simulink model "Target_Control_System"  (R2021b)
settings: Solver=FixedStepDiscrete  StartTime=0.0  StopTime=5  RelTol=1e-3
PreLoadFcn:
  | RTWConfigurationCB('preloadfcn', bdroot);
PostLoadFcn:
  | load('configuration/data_struct.mat');
  | load('configuration/fluxMaps_propMotor.mat');
  | load('configuration/parameterInit_PROP.mat');
  | load('configuration/parameterInit_PUMP.mat');
  | load('configuration/parameterInit_PITCH.mat');
  | load('configuration/parameterInit_TILT.mat');
  | %load('configuration/base_workspace_signal_definition.mat');
  | %load('resolvedatastores_to_baseworkspace_for_faster_simulation.mat');
model workspace (MAT data in the model file):
  SIMULATION_OPTIONS : Simulink.Parameter (value not decoded)
  TARGET_CODE_GEN : Simulink.Parameter (value not decoded)
  TCS_SAMPLE_FREQ_HZ : Simulink.Parameter (value not decoded)
symbols that are objects in the model workspace (value not decoded): TARGET_CODE_GEN, TCS_SAMPLE_FREQ_HZ
undefined symbols (not defined in the file): A_DQ_REF_LPF_INIT__PITCH, A_DQ_REF_LPF_INIT__PROP, A_DQ_REF_LPF_INIT__PUMP, A_DQ_REF_LPF_INIT__TILT, A_OBSERVER_CONFIDENCE_INIT__PITCH, A_OBSERVER_CONFIDENCE_INIT__PROP, A_OBSERVER_CONFIDENCE_INIT__PUMP, A_OBSERVER_CONFIDENCE_INIT__TILT, ACTUATOR_MAX_ANGLE_TRIP__PITCH, ACTUATOR_MIN_ANGLE_TRIP__PITCH, ACTUATOR_POS_SENSOR_INV_DIRECTION__PITCH, ACTUATOR_POS_SENSOR_INV_DIRECTION__TILT, ACTUATOR_POS_SENSOR_OFFSET__PITCH, ACTUATOR_POS_SENSOR_OFFSET__TILT, ADC_scaler1_baseaddr_TILT, ADC_SCALER_FLOAT_TO_FIXPOINT_EXPANSION, ANGLE_ELEC_FROM_SENSOR_OFFSET_INIT__PITCH, ANGLE_ELEC_FROM_SENSOR_OFFSET_INIT__PROP, ANGLE_ELEC_FROM_SENSOR_OFFSET_INIT__PUMP, ANGLE_ELEC_FROM_SENSOR_OFFSET_INIT__TILT, AUTO_CLEAR_FAULTS_ENABLED__PITCH, AUTO_CLEAR_FAULTS_ENABLED__PROP, AUTO_CLEAR_FAULTS_ENABLED__PUMP, AUTO_CLEAR_FAULTS_ENABLED__TILT, AUTO_CLEAR_FAULTS_WAIT_TICKS__PITCH, AUTO_CLEAR_FAULTS_WAIT_TICKS__PROP, AUTO_CLEAR_FAULTS_WAIT_TICKS__PUMP, AUTO_CLEAR_FAULTS_WAIT_TICKS__TILT, AUTO_I_ZERO_IDLE_TICKS__PITCH, AUTO_I_ZERO_IDLE_TICKS__PROP, AUTO_I_ZERO_IDLE_TICKS__PUMP, AUTO_I_ZERO_IDLE_TICKS__TILT, AUTO_I_ZERO_OFFSET_IDC_THRESHOLD__PITCH, AUTO_I_ZERO_OFFSET_IDC_THRESHOLD__PROP, AUTO_I_ZERO_OFFSET_IDC_THRESHOLD__PUMP, AUTO_I_ZERO_OFFSET_IDC_THRESHOLD__TILT, AUTO_I_ZERO_OFFSET_IPH_THRESHOLD__PITCH, AUTO_I_ZERO_OFFSET_IPH_THRESHOLD__PROP, AUTO_I_ZERO_OFFSET_IPH_THRESHOLD__PUMP, AUTO_I_ZERO_OFFSET_IPH_THRESHOLD__TILT, AUTO_SENSORLESS_SWITCHOVER_DISABLE_OMEGA, AUTO_SENSORLESS_SWITCHOVER_ENABLE_OMEGA, AUTO_SENSORLESS_SWITCHOVER_MIN_CONFIDENCE, AUXILIARY_PROTECTION_UNIT_BASEADDR__TILT, blanking_max_error_omega_INIT_PITCH, blanking_max_error_omega_INIT_TILT, blanking_max_error_position_INIT_PITCH, blanking_max_error_position_INIT_TILT, BRUTE_START_I_Q_REF_RAMP_SPEED__PITCH, BRUTE_START_I_Q_REF_RAMP_SPEED__PROP, BRUTE_START_I_Q_REF_RAMP_SPEED__PUMP, BRUTE_START_I_Q_REF_RAMP_SPEED__TILT, CONTROL_LOOP_DT_INIT__PITCH, CONTROL_LOOP_DT_INIT__PROP, CONTROL_LOOP_DT_INIT__PUMP, CONTROL_LOOP_DT_INIT__TILT, CORRECTION_FILTER_SCALE__PITCH, CORRECTION_FILTER_SCALE__PROP, CORRECTION_FILTER_SCALE__PUMP, CORRECTION_FILTER_SCALE__TILT ... (+458)
libraries: simulink x178, Reusables_Lib x24
(part 24 of 47)

== system Target_Control_System/Target_Control_System/Simulation Controls/Simulation Data Store Initialization/setupIirFilters(&oTilt)/computeCoefficientsButter()1 ==
  fCutoffFrequencyHz : Inport  OutDataTypeStr=single
  dSampleFrequencyHz : Inport  Port=2  OutDataTypeStr=single
  Add : Sum  Inputs=+++  OutDataTypeStr=double
  Add1 : Sum  Inputs=-+
  Add2 : Sum  Inputs=+-+  OutDataTypeStr=double
  Constant : Constant  Value=0.0008  OutDataTypeStr=single  SampleTime=-1
  Constant1 : Constant  Value=0.45  OutDataTypeStr=single  SampleTime=-1
  Constant{5,7,9..10} (4 alike) : Constant  SampleTime=-1
  Constant2 : Constant  Value=pi  OutDataTypeStr=double  SampleTime=-1
  Constant3 : Constant  OutDataTypeStr=double  SampleTime=-1
  Constant4 : Constant  Value=sqrt(2)  OutDataTypeStr=double  SampleTime=-1
  Constant6 : Constant  OutDataTypeStr=double  SampleTime=-1
  Constant8 : Constant  Value=2  SampleTime=-1
  Data Type Conversion : DataTypeConversion  OutDataTypeStr=double
  Divide : Product  Inputs=**  OutDataTypeStr=single
  Divide1 : Product  Inputs=**  OutDataTypeStr=single
  Divide{3,5..6,8,10..11} (6 alike) : Product  Inputs=**  OutDataTypeStr=double
  Divide2 : Product  Inputs=*/  OutDataTypeStr=double
  Divide4 : Product  Inputs=*/  OutDataTypeStr=double
  Divide7 : Product  Inputs=*/  OutDataTypeStr=double
  Divide9 : Product  Inputs=***  OutDataTypeStr=double
  Gain : Gain  Gain=2  OutDataTypeStr=double
  Gain1 : Gain  Gain=-1  OutDataTypeStr=double
  Gain2 : Gain  Gain=-1  OutDataTypeStr=double
  Gain3 : Gain  Gain=-1  OutDataTypeStr=double
  Mux : Mux  Inputs=6
  Saturation Dynamic : simulink/Discontinuities/Saturation Dynamic  OutMin=[]  OutMax=[]  OutDataTypeStr=Inherit: Same as second input  OutDataType=fixdt(1, 16)  OutScaling=2^-10  DoSatur=off
  Tan : Trigonometry  Operator=tan
  dpOutArray : Outport
  fCutoffFrequencyHz_out : Outport  Port=2
  wires:
  Saturation Dynamic/1 -> Data Type Conversion/1, fCutoffFrequencyHz_out/1  "fCutoffFrequencyHz"
  Data Type Conversion/1 -> Divide2/1
  Constant10/1 -> Mux/4
  [dA2] -> Gain3/1
  Gain3/1 -> Mux/6
  [dA1] -> Gain2/1
  Gain2/1 -> Mux/5
  [dB2] -> Mux/3
  [dB1] -> Mux/2
  [dB0] -> Mux/1
  Divide11/1 -> [dA2]
  Gain1/1 -> Divide11/2
  Add2/1 -> Gain1/1
  Constant9/1 -> Add2/3
  Divide10/1 -> Add2/2
  [kdQ] -> Divide10/2
  Constant7/1 -> Add1/1
  Divide8/1 -> Add1/2, Add2/1
  Divide9/1 -> [dA1]
  Constant8/1 -> Divide9/3
  Add1/1 -> Divide9/2
  [kdIta] -> Divide8/1, Divide8/2, Divide10/1
  Gain/1 -> [dB1]
  Divide7/1 -> [dB0], Gain/1, [dB2], Divide9/1, Divide11/1
  Add/1 -> Divide7/2
  Constant6/1 -> Divide7/1
  Constant5/1 -> Add/3
  Divide5/1 -> Add/2
  Divide6/1 -> Add/1
  [kdQ] -> Divide5/2
  [kdIta] -> Divide5/1, Divide6/1, Divide6/2
  Mux/1 -> dpOutArray/1
  Constant4/1 -> [kdQ]
  Divide4/1 -> [kdIta]
  Constant3/1 -> Divide4/1
  Tan/1 -> Divide4/2
  Divide3/1 -> Tan/1
  Constant2/1 -> Divide3/2
  Divide2/1 -> Divide3/1  "dFf"
  Constant/1 -> Divide/2
  fCutoffFrequencyHz/1 -> Saturation Dynamic/2  "fCutoffFrequencyHz"
  Divide1/1 -> Saturation Dynamic/1
  dSampleFrequencyHz/1 -> Divide1/2, Divide2/2, Divide/1
  Constant1/1 -> Divide1/1
  Divide/1 -> Saturation Dynamic/3

== system Target_Control_System/Target_Control_System/Simulation Controls/Simulation Data Store Initialization/setupIirFilters(&oTilt)/computeCoefficientsButter()2 ==
  fCutoffFrequencyHz : Inport  OutDataTypeStr=single
  dSampleFrequencyHz : Inport  Port=2  OutDataTypeStr=single
  Add : Sum  Inputs=+++  OutDataTypeStr=double
  Add1 : Sum  Inputs=-+
  Add2 : Sum  Inputs=+-+  OutDataTypeStr=double
  Constant : Constant  Value=0.0008  OutDataTypeStr=single  SampleTime=-1
  Constant1 : Constant  Value=0.45  OutDataTypeStr=single  SampleTime=-1
  Constant{5,7,9..10} (4 alike) : Constant  SampleTime=-1
  Constant2 : Constant  Value=pi  OutDataTypeStr=double  SampleTime=-1
  Constant3 : Constant  OutDataTypeStr=double  SampleTime=-1
  Constant4 : Constant  Value=sqrt(2)  OutDataTypeStr=double  SampleTime=-1
  Constant6 : Constant  OutDataTypeStr=double  SampleTime=-1
  Constant8 : Constant  Value=2  SampleTime=-1
  Data Type Conversion : DataTypeConversion  OutDataTypeStr=double
  Divide : Product  Inputs=**  OutDataTypeStr=single
  Divide1 : Product  Inputs=**  OutDataTypeStr=single
  Divide{3,5..6,8,10..11} (6 alike) : Product  Inputs=**  OutDataTypeStr=double
  Divide2 : Product  Inputs=*/  OutDataTypeStr=double
  Divide4 : Product  Inputs=*/  OutDataTypeStr=double
  Divide7 : Product  Inputs=*/  OutDataTypeStr=double
  Divide9 : Product  Inputs=***  OutDataTypeStr=double
  Gain : Gain  Gain=2  OutDataTypeStr=double
  Gain1 : Gain  Gain=-1  OutDataTypeStr=double
  Gain2 : Gain  Gain=-1  OutDataTypeStr=double
  Gain3 : Gain  Gain=-1  OutDataTypeStr=double
  Mux : Mux  Inputs=6
  Saturation Dynamic : simulink/Discontinuities/Saturation Dynamic  OutMin=[]  OutMax=[]  OutDataTypeStr=Inherit: Same as second input  OutDataType=fixdt(1, 16)  OutScaling=2^-10  DoSatur=off
  Tan : Trigonometry  Operator=tan
  dpOutArray : Outport
  fCutoffFrequencyHz_out : Outport  Port=2
  wires:
  Saturation Dynamic/1 -> Data Type Conversion/1, fCutoffFrequencyHz_out/1  "fCutoffFrequencyHz"
  Data Type Conversion/1 -> Divide2/1
  Constant10/1 -> Mux/4
  [dA2] -> Gain3/1
  Gain3/1 -> Mux/6
  [dA1] -> Gain2/1
  Gain2/1 -> Mux/5
  [dB2] -> Mux/3
  [dB1] -> Mux/2
  [dB0] -> Mux/1
  Divide11/1 -> [dA2]
  Gain1/1 -> Divide11/2
  Add2/1 -> Gain1/1
  Constant9/1 -> Add2/3
  Divide10/1 -> Add2/2
  [kdQ] -> Divide10/2
  Constant7/1 -> Add1/1
  Divide8/1 -> Add1/2, Add2/1
  Divide9/1 -> [dA1]
  Constant8/1 -> Divide9/3
  Add1/1 -> Divide9/2
  [kdIta] -> Divide8/1, Divide8/2, Divide10/1
  Gain/1 -> [dB1]
  Divide7/1 -> [dB0], Gain/1, [dB2], Divide9/1, Divide11/1
  Add/1 -> Divide7/2
  Constant6/1 -> Divide7/1
  Constant5/1 -> Add/3
  Divide5/1 -> Add/2
  Divide6/1 -> Add/1
  [kdQ] -> Divide5/2
  [kdIta] -> Divide5/1, Divide6/1, Divide6/2
  Mux/1 -> dpOutArray/1
  Constant4/1 -> [kdQ]
  Divide4/1 -> [kdIta]
  Constant3/1 -> Divide4/1
  Tan/1 -> Divide4/2
  Divide3/1 -> Tan/1
  Constant2/1 -> Divide3/2
  Divide2/1 -> Divide3/1  "dFf"
  Constant/1 -> Divide/2
  fCutoffFrequencyHz/1 -> Saturation Dynamic/2  "fCutoffFrequencyHz"
  Divide1/1 -> Saturation Dynamic/1
  dSampleFrequencyHz/1 -> Divide1/2, Divide2/2, Divide/1
  Constant1/1 -> Divide1/1
  Divide/1 -> Saturation Dynamic/3

== system Target_Control_System/Target_Control_System/Simulation Controls/Simulation Data Store Initialization/setupIirFilters(&oTilt)/softwareIirFilterInitialize() ==
  fFreq3db : Inport
  fFreqSample : Inport  Port=2
  Constant : Constant  OutDataTypeStr=single  SampleTime=-1
  Constant1 : Constant  Value=0  OutDataTypeStr=single  SampleTime=-1
  Data Store Write : DataStoreWrite  DataStoreName=oTilt  DataStoreElements=oTilt.oMot_.oState_.oMotorAccelerationFilterStage2_.afConstantsA_.h0  IndexOptions=Index vector (dialog)  Indices=1  OutputSizes=1
  Data Store Write1 : DataStoreWrite  DataStoreName=oTilt  DataStoreElements=oTilt.oMot_.oState_.oMotorAccelerationFilterStage2_.afConstantsA_.h1  IndexOptions=Index vector (dialog)  Indices=1  OutputSizes=1
  Data Store Write10 : DataStoreWrite  DataStoreName=oTilt  DataStoreElements=oTilt.oMot_.oState_.oMotorAccelerationFilterStage2_.fFilterOutput_  IndexOptions=Index vector (dialog)  Indices=1  OutputSizes=1
  Data Store Write2 : DataStoreWrite  DataStoreName=oTilt  DataStoreElements=oTilt.oMot_.oState_.oMotorAccelerationFilterStage2_.afConstantsA_.h2  IndexOptions=Index vector (dialog)  Indices=1  OutputSizes=1
  Data Store Write3 : DataStoreWrite  DataStoreName=oTilt  DataStoreElements=oTilt.oMot_.oState_.oMotorAccelerationFilterStage2_.afConstantsB_.h2  IndexOptions=Index vector (dialog)  Indices=1  OutputSizes=1
  Data Store Write4 : DataStoreWrite  DataStoreName=oTilt  DataStoreElements=oTilt.oMot_.oState_.oMotorAccelerationFilterStage2_.afConstantsB_.h1  IndexOptions=Index vector (dialog)  Indices=1  OutputSizes=1
  Data Store Write5 : DataStoreWrite  DataStoreName=oTilt  DataStoreElements=oTilt.oMot_.oState_.oMotorAccelerationFilterStage2_.afConstantsB_.h0  IndexOptions=Index vector (dialog)  Indices=1  OutputSizes=1
  Data Store Write6 : DataStoreWrite  DataStoreName=oTilt  DataStoreElements=oTilt.oMot_.oState_.oMotorAccelerationFilterStage2_.afPreviousInputs_.h0  IndexOptions=Index vector (dialog)  Indices=1  OutputSizes=1
  Data Store Write7 : DataStoreWrite  DataStoreName=oTilt  DataStoreElements=oTilt.oMot_.oState_.oMotorAccelerationFilterStage2_.afPreviousInputs_.h1  IndexOptions=Index vector (dialog)  Indices=1  OutputSizes=1
  Data Store Write8 : DataStoreWrite  DataStoreName=oTilt  DataStoreElements=oTilt.oMot_.oState_.oMotorAccelerationFilterStage2_.afPreviousOutputs_.h0  IndexOptions=Index vector (dialog)  Indices=1  OutputSizes=1
  Data Store Write9 : DataStoreWrite  DataStoreName=oTilt  DataStoreElements=oTilt.oMot_.oState_.oMotorAccelerationFilterStage2_.afPreviousOutputs_.h1  IndexOptions=Index vector (dialog)  Indices=1  OutputSizes=1
  Data Type Conversion{1..5} (5 alike) : DataTypeConversion  OutDataTypeStr=single
  Demux : Demux  Outputs=6
  Divide : Product  Inputs=*/  OutDataTypeStr=single
  computeCoefficientsButter() : Subsystem
  fActualFrequencyHz : Outport
  wires:
  Data Type Conversion5/1 -> Data Store Write2/1
  Data Type Conversion4/1 -> Data Store Write1/1
  Data Type Conversion3/1 -> Data Store Write3/1
  Data Type Conversion1/1 -> Data Store Write4/1
  Data Type Conversion2/1 -> Data Store Write5/1
  fFreqSample/1 -> computeCoefficientsButter()/2(dSampleFrequencyHz)
  Constant1/1 -> Data Store Write6/1, Data Store Write7/1, Data Store Write9/1, Data Store Write10/1, Data Store Write8/1
  Demux/1 -> Data Type Conversion2/1
  Demux/2 -> Data Type Conversion1/1
  Constant/1 -> Divide/1
  Divide/1 -> Data Store Write/1
  Demux/4 -> Divide/2
  Demux/3 -> Data Type Conversion3/1
  Demux/5 -> Data Type Conversion4/1
  Demux/6 -> Data Type Conversion5/1
  computeCoefficientsButter()/1(dpOutArray) -> Demux/1
  fFreq3db/1 -> computeCoefficientsButter()/1(fCutoffFrequencyHz)
  computeCoefficientsButter()/2(fFreq3db) -> fActualFrequencyHz/1

== system Target_Control_System/Target_Control_System/Simulation Controls/Simulation Data Store Initialization/setupIirFilters()/computeCoefficientsButter() ==
  fCutoffFrequencyHz : Inport  OutDataTypeStr=single
  dSampleFrequencyHz : Inport  Port=2  OutDataTypeStr=single
  Add : Sum  Inputs=+++  OutDataTypeStr=double
  Add1 : Sum  Inputs=-+
  Add2 : Sum  Inputs=+-+  OutDataTypeStr=double
  Constant : Constant  Value=0.0008  OutDataTypeStr=single  SampleTime=-1
  Constant1 : Constant  Value=0.45  OutDataTypeStr=single  SampleTime=-1
  Constant{5,7,9..10} (4 alike) : Constant  SampleTime=-1
  Constant2 : Constant  Value=pi  OutDataTypeStr=double  SampleTime=-1
  Constant3 : Constant  OutDataTypeStr=double  SampleTime=-1
  Constant4 : Constant  Value=sqrt(2)  OutDataTypeStr=double  SampleTime=-1
  Constant6 : Constant  OutDataTypeStr=double  SampleTime=-1
  Constant8 : Constant  Value=2  SampleTime=-1
  Data Type Conversion : DataTypeConversion  OutDataTypeStr=double
  Divide : Product  Inputs=**  OutDataTypeStr=single
  Divide1 : Product  Inputs=**  OutDataTypeStr=single
  Divide{3,5..6,8,10..11} (6 alike) : Product  Inputs=**  OutDataTypeStr=double
  Divide2 : Product  Inputs=*/  OutDataTypeStr=double
  Divide4 : Product  Inputs=*/  OutDataTypeStr=double
  Divide7 : Product  Inputs=*/  OutDataTypeStr=double
  Divide9 : Product  Inputs=***  OutDataTypeStr=double
  Gain : Gain  Gain=2  OutDataTypeStr=double
  Gain1 : Gain  Gain=-1  OutDataTypeStr=double
  Gain2 : Gain  Gain=-1  OutDataTypeStr=double
  Gain3 : Gain  Gain=-1  OutDataTypeStr=double
  Mux : Mux  Inputs=6
  Saturation Dynamic : simulink/Discontinuities/Saturation Dynamic  OutMin=[]  OutMax=[]  OutDataTypeStr=Inherit: Same as second input  OutDataType=fixdt(1, 16)  OutScaling=2^-10  DoSatur=off
  Tan : Trigonometry  Operator=tan
  dpOutArray : Outport
  fCutoffFrequencyHz_out : Outport  Port=2
  wires:
  Saturation Dynamic/1 -> Data Type Conversion/1, fCutoffFrequencyHz_out/1  "fCutoffFrequencyHz"
  Data Type Conversion/1 -> Divide2/1
  Constant10/1 -> Mux/4
  [dA2] -> Gain3/1
  Gain3/1 -> Mux/6
  [dA1] -> Gain2/1
  Gain2/1 -> Mux/5
  [dB2] -> Mux/3
  [dB1] -> Mux/2
  [dB0] -> Mux/1
  Divide11/1 -> [dA2]
  Gain1/1 -> Divide11/2
  Add2/1 -> Gain1/1
  Constant9/1 -> Add2/3
  Divide10/1 -> Add2/2
  [kdQ] -> Divide10/2
  Constant7/1 -> Add1/1
  Divide8/1 -> Add1/2, Add2/1
  Divide9/1 -> [dA1]
  Constant8/1 -> Divide9/3
  Add1/1 -> Divide9/2
  [kdIta] -> Divide8/1, Divide8/2, Divide10/1
  Gain/1 -> [dB1]
  Divide7/1 -> [dB0], Gain/1, [dB2], Divide9/1, Divide11/1
  Add/1 -> Divide7/2
  Constant6/1 -> Divide7/1
  Constant5/1 -> Add/3
  Divide5/1 -> Add/2
  Divide6/1 -> Add/1
  [kdQ] -> Divide5/2
  [kdIta] -> Divide5/1, Divide6/1, Divide6/2
  Mux/1 -> dpOutArray/1
  Constant4/1 -> [kdQ]
  Divide4/1 -> [kdIta]
  Constant3/1 -> Divide4/1
  Tan/1 -> Divide4/2
  Divide3/1 -> Tan/1
  Constant2/1 -> Divide3/2
  Divide2/1 -> Divide3/1  "dFf"
  Constant/1 -> Divide/2
  fCutoffFrequencyHz/1 -> Saturation Dynamic/2  "fCutoffFrequencyHz"
  Divide1/1 -> Saturation Dynamic/1
  dSampleFrequencyHz/1 -> Divide1/2, Divide2/2, Divide/1
  Constant1/1 -> Divide1/1
  Divide/1 -> Saturation Dynamic/3

== system Target_Control_System/Target_Control_System/Simulation Controls/Simulation Data Store Initialization/setupIirFilters()/computeCoefficientsButter()1 ==
  fCutoffFrequencyHz : Inport  OutDataTypeStr=single
  dSampleFrequencyHz : Inport  Port=2  OutDataTypeStr=single
  Add : Sum  Inputs=+++  OutDataTypeStr=double
  Add1 : Sum  Inputs=-+
  Add2 : Sum  Inputs=+-+  OutDataTypeStr=double
  Constant : Constant  Value=0.0008  OutDataTypeStr=single  SampleTime=-1
  Constant1 : Constant  Value=0.45  OutDataTypeStr=single  SampleTime=-1
  Constant{5,7,9..10} (4 alike) : Constant  SampleTime=-1
  Constant2 : Constant  Value=pi  OutDataTypeStr=double  SampleTime=-1
  Constant3 : Constant  OutDataTypeStr=double  SampleTime=-1
  Constant4 : Constant  Value=sqrt(2)  OutDataTypeStr=double  SampleTime=-1
  Constant6 : Constant  OutDataTypeStr=double  SampleTime=-1
  Constant8 : Constant  Value=2  SampleTime=-1
  Data Type Conversion : DataTypeConversion  OutDataTypeStr=double
  Divide : Product  Inputs=**  OutDataTypeStr=single
  Divide1 : Product  Inputs=**  OutDataTypeStr=single
  Divide{3,5..6,8,10..11} (6 alike) : Product  Inputs=**  OutDataTypeStr=double
  Divide2 : Product  Inputs=*/  OutDataTypeStr=double
  Divide4 : Product  Inputs=*/  OutDataTypeStr=double
  Divide7 : Product  Inputs=*/  OutDataTypeStr=double
  Divide9 : Product  Inputs=***  OutDataTypeStr=double
  Gain : Gain  Gain=2  OutDataTypeStr=double
  Gain1 : Gain  Gain=-1  OutDataTypeStr=double
  Gain2 : Gain  Gain=-1  OutDataTypeStr=double
  Gain3 : Gain  Gain=-1  OutDataTypeStr=double
  Mux : Mux  Inputs=6
  Saturation Dynamic : simulink/Discontinuities/Saturation Dynamic  OutMin=[]  OutMax=[]  OutDataTypeStr=Inherit: Same as second input  OutDataType=fixdt(1, 16)  OutScaling=2^-10  DoSatur=off
  Tan : Trigonometry  Operator=tan
  dpOutArray : Outport
  fCutoffFrequencyHz_out : Outport  Port=2
  wires:
  Saturation Dynamic/1 -> Data Type Conversion/1, fCutoffFrequencyHz_out/1  "fCutoffFrequencyHz"
  Data Type Conversion/1 -> Divide2/1
  Constant10/1 -> Mux/4
  [dA2] -> Gain3/1
  Gain3/1 -> Mux/6
  [dA1] -> Gain2/1
  Gain2/1 -> Mux/5
  [dB2] -> Mux/3
  [dB1] -> Mux/2
  [dB0] -> Mux/1
  Divide11/1 -> [dA2]
  Gain1/1 -> Divide11/2
  Add2/1 -> Gain1/1
  Constant9/1 -> Add2/3
  Divide10/1 -> Add2/2
  [kdQ] -> Divide10/2
  Constant7/1 -> Add1/1
  Divide8/1 -> Add1/2, Add2/1
  Divide9/1 -> [dA1]
  Constant8/1 -> Divide9/3
  Add1/1 -> Divide9/2
  [kdIta] -> Divide8/1, Divide8/2, Divide10/1
  Gain/1 -> [dB1]
  Divide7/1 -> [dB0], Gain/1, [dB2], Divide9/1, Divide11/1
  Add/1 -> Divide7/2
  Constant6/1 -> Divide7/1
  Constant5/1 -> Add/3
  Divide5/1 -> Add/2
  Divide6/1 -> Add/1
  [kdQ] -> Divide5/2
  [kdIta] -> Divide5/1, Divide6/1, Divide6/2
  Mux/1 -> dpOutArray/1
  Constant4/1 -> [kdQ]
  Divide4/1 -> [kdIta]
  Constant3/1 -> Divide4/1
  Tan/1 -> Divide4/2
  Divide3/1 -> Tan/1
  Constant2/1 -> Divide3/2
  Divide2/1 -> Divide3/1  "dFf"
  Constant/1 -> Divide/2
  fCutoffFrequencyHz/1 -> Saturation Dynamic/2  "fCutoffFrequencyHz"
  Divide1/1 -> Saturation Dynamic/1
  dSampleFrequencyHz/1 -> Divide1/2, Divide2/2, Divide/1
  Constant1/1 -> Divide1/1
  Divide/1 -> Saturation Dynamic/3

== system Target_Control_System/Target_Control_System/Simulation Controls/Simulation Data Store Initialization/setupIirFilters()/computeCoefficientsButter()2 ==
  fCutoffFrequencyHz : Inport  OutDataTypeStr=single
  dSampleFrequencyHz : Inport  Port=2  OutDataTypeStr=single
  Add : Sum  Inputs=+++  OutDataTypeStr=double
  Add1 : Sum  Inputs=-+
  Add2 : Sum  Inputs=+-+  OutDataTypeStr=double
  Constant : Constant  Value=0.0008  OutDataTypeStr=single  SampleTime=-1
  Constant1 : Constant  Value=0.45  OutDataTypeStr=single  SampleTime=-1
  Constant{5,7,9..10} (4 alike) : Constant  SampleTime=-1
  Constant2 : Constant  Value=pi  OutDataTypeStr=double  SampleTime=-1
  Constant3 : Constant  OutDataTypeStr=double  SampleTime=-1
  Constant4 : Constant  Value=sqrt(2)  OutDataTypeStr=double  SampleTime=-1
  Constant6 : Constant  OutDataTypeStr=double  SampleTime=-1
  Constant8 : Constant  Value=2  SampleTime=-1
  Data Type Conversion : DataTypeConversion  OutDataTypeStr=double
  Divide : Product  Inputs=**  OutDataTypeStr=single
  Divide1 : Product  Inputs=**  OutDataTypeStr=single
  Divide{3,5..6,8,10..11} (6 alike) : Product  Inputs=**  OutDataTypeStr=double
  Divide2 : Product  Inputs=*/  OutDataTypeStr=double
  Divide4 : Product  Inputs=*/  OutDataTypeStr=double
  Divide7 : Product  Inputs=*/  OutDataTypeStr=double
  Divide9 : Product  Inputs=***  OutDataTypeStr=double
  Gain : Gain  Gain=2  OutDataTypeStr=double
  Gain1 : Gain  Gain=-1  OutDataTypeStr=double
  Gain2 : Gain  Gain=-1  OutDataTypeStr=double
  Gain3 : Gain  Gain=-1  OutDataTypeStr=double
  Mux : Mux  Inputs=6
  Saturation Dynamic : simulink/Discontinuities/Saturation Dynamic  OutMin=[]  OutMax=[]  OutDataTypeStr=Inherit: Same as second input  OutDataType=fixdt(1, 16)  OutScaling=2^-10  DoSatur=off
  Tan : Trigonometry  Operator=tan
  dpOutArray : Outport
  fCutoffFrequencyHz_out : Outport  Port=2
  wires:
  Saturation Dynamic/1 -> Data Type Conversion/1, fCutoffFrequencyHz_out/1  "fCutoffFrequencyHz"
  Data Type Conversion/1 -> Divide2/1
  Constant10/1 -> Mux/4
  [dA2] -> Gain3/1
  Gain3/1 -> Mux/6
  [dA1] -> Gain2/1
  Gain2/1 -> Mux/5
  [dB2] -> Mux/3
  [dB1] -> Mux/2
  [dB0] -> Mux/1
  Divide11/1 -> [dA2]
  Gain1/1 -> Divide11/2
  Add2/1 -> Gain1/1
  Constant9/1 -> Add2/3
  Divide10/1 -> Add2/2
  [kdQ] -> Divide10/2
  Constant7/1 -> Add1/1
  Divide8/1 -> Add1/2, Add2/1
  Divide9/1 -> [dA1]
  Constant8/1 -> Divide9/3
  Add1/1 -> Divide9/2
  [kdIta] -> Divide8/1, Divide8/2, Divide10/1
  Gain/1 -> [dB1]
  Divide7/1 -> [dB0], Gain/1, [dB2], Divide9/1, Divide11/1
  Add/1 -> Divide7/2
  Constant6/1 -> Divide7/1
  Constant5/1 -> Add/3
  Divide5/1 -> Add/2
  Divide6/1 -> Add/1
  [kdQ] -> Divide5/2
  [kdIta] -> Divide5/1, Divide6/1, Divide6/2
  Mux/1 -> dpOutArray/1
  Constant4/1 -> [kdQ]
  Divide4/1 -> [kdIta]
  Constant3/1 -> Divide4/1
  Tan/1 -> Divide4/2
  Divide3/1 -> Tan/1
  Constant2/1 -> Divide3/2
  Divide2/1 -> Divide3/1  "dFf"
  Constant/1 -> Divide/2
  fCutoffFrequencyHz/1 -> Saturation Dynamic/2  "fCutoffFrequencyHz"
  Divide1/1 -> Saturation Dynamic/1
  dSampleFrequencyHz/1 -> Divide1/2, Divide2/2, Divide/1
  Constant1/1 -> Divide1/1
  Divide/1 -> Saturation Dynamic/3

== system Target_Control_System/Target_Control_System/Simulation Controls/Simulation Data Store Initialization/setupIirFilters()/softwareIirFilterInitialize() ==
  fFreq3db : Inport
  fFreqSample : Inport  Port=2
  Constant : Constant  OutDataTypeStr=single  SampleTime=-1
  Constant1 : Constant  Value=0  OutDataTypeStr=single  SampleTime=-1
  Data Store Write : DataStoreWrite  DataStoreName=oPitch  DataStoreElements=oPitch.oMot_.oState_.oMotorAccelerationFilterStage2_.afConstantsA_.h0  IndexOptions=Index vector (dialog)  Indices=1  OutputSizes=1
  Data Store Write1 : DataStoreWrite  DataStoreName=oPitch  DataStoreElements=oPitch.oMot_.oState_.oMotorAccelerationFilterStage2_.afConstantsA_.h1  IndexOptions=Index vector (dialog)  Indices=1  OutputSizes=1
  Data Store Write10 : DataStoreWrite  DataStoreName=oPitch  DataStoreElements=oPitch.oMot_.oState_.oMotorAccelerationFilterStage2_.fFilterOutput_  IndexOptions=Index vector (dialog)  Indices=1  OutputSizes=1
  Data Store Write2 : DataStoreWrite  DataStoreName=oPitch  DataStoreElements=oPitch.oMot_.oState_.oMotorAccelerationFilterStage2_.afConstantsA_.h2  IndexOptions=Index vector (dialog)  Indices=1  OutputSizes=1
  Data Store Write3 : DataStoreWrite  DataStoreName=oPitch  DataStoreElements=oPitch.oMot_.oState_.oMotorAccelerationFilterStage2_.afConstantsB_.h2  IndexOptions=Index vector (dialog)  Indices=1  OutputSizes=1
  Data Store Write4 : DataStoreWrite  DataStoreName=oPitch  DataStoreElements=oPitch.oMot_.oState_.oMotorAccelerationFilterStage2_.afConstantsB_.h1  IndexOptions=Index vector (dialog)  Indices=1  OutputSizes=1
  Data Store Write5 : DataStoreWrite  DataStoreName=oPitch  DataStoreElements=oPitch.oMot_.oState_.oMotorAccelerationFilterStage2_.afConstantsB_.h0  IndexOptions=Index vector (dialog)  Indices=1  OutputSizes=1
  Data Store Write6 : DataStoreWrite  DataStoreName=oPitch  DataStoreElements=oPitch.oMot_.oState_.oMotorAccelerationFilterStage2_.afPreviousInputs_.h0  IndexOptions=Index vector (dialog)  Indices=1  OutputSizes=1
  Data Store Write7 : DataStoreWrite  DataStoreName=oPitch  DataStoreElements=oPitch.oMot_.oState_.oMotorAccelerationFilterStage2_.afPreviousInputs_.h1  IndexOptions=Index vector (dialog)  Indices=1  OutputSizes=1
  Data Store Write8 : DataStoreWrite  DataStoreName=oPitch  DataStoreElements=oPitch.oMot_.oState_.oMotorAccelerationFilterStage2_.afPreviousOutputs_.h0  IndexOptions=Index vector (dialog)  Indices=1  OutputSizes=1
  Data Store Write9 : DataStoreWrite  DataStoreName=oPitch  DataStoreElements=oPitch.oMot_.oState_.oMotorAccelerationFilterStage2_.afPreviousOutputs_.h1  IndexOptions=Index vector (dialog)  Indices=1  OutputSizes=1
  Data Type Conversion{1..5} (5 alike) : DataTypeConversion  OutDataTypeStr=single
  Demux : Demux  Outputs=6
  Divide : Product  Inputs=*/  OutDataTypeStr=single
  computeCoefficientsButter() : Subsystem
  fActualFrequencyHz : Outport
  wires:
  Data Type Conversion5/1 -> Data Store Write2/1
  Data Type Conversion4/1 -> Data Store Write1/1
  Data Type Conversion3/1 -> Data Store Write3/1
  Data Type Conversion1/1 -> Data Store Write4/1
  Data Type Conversion2/1 -> Data Store Write5/1
  fFreqSample/1 -> computeCoefficientsButter()/2(dSampleFrequencyHz)
  Constant1/1 -> Data Store Write6/1, Data Store Write7/1, Data Store Write9/1, Data Store Write10/1, Data Store Write8/1
  Demux/1 -> Data Type Conversion2/1
  Demux/2 -> Data Type Conversion1/1
  Constant/1 -> Divide/1
  Divide/1 -> Data Store Write/1
  Demux/4 -> Divide/2
  Demux/3 -> Data Type Conversion3/1
  Demux/5 -> Data Type Conversion4/1
  Demux/6 -> Data Type Conversion5/1
  computeCoefficientsButter()/1(dpOutArray) -> Demux/1
  fFreq3db/1 -> computeCoefficientsButter()/1(fCutoffFrequencyHz)
  computeCoefficientsButter()/2(fFreq3db) -> fActualFrequencyHz/1

== system Target_Control_System/Target_Control_System/Simulation Controls/Simulation Data Store Initialization/setupObserver()/updateObserver()_pitch ==
  oIsr_.oParam_.fControlLoopDt_ : Inport
  fObserverLoopFilterBandwidthHz_ : Inport  Port=2
  Constant : Constant  Value=15*2*pi  OutDataTypeStr=single  SampleTime=-1
  Constant1 : Constant  Value=8*2*pi  OutDataTypeStr=single  SampleTime=-1
  Constant2 : Constant  Value=2*pi  OutDataTypeStr=single  SampleTime=-1
  Constant3 : Constant  Value=500  OutDataTypeStr=single  SampleTime=-1
  Constant4 : Constant  Value=20  OutDataTypeStr=single  SampleTime=-1
  Constant5 : Constant  Value=100*2*pi  OutDataTypeStr=single  SampleTime=-1
  Constant6 : Constant  Value=4*2*pi  OutDataTypeStr=single  SampleTime=-1
  Constant7 : Constant  Value=0.0625  OutDataTypeStr=single  SampleTime=-1
  Data Store Write : DataStoreWrite  DataStoreName=oPitch  DataStoreElements=oPitch.oIsr_.oParam_.fALpf4hpfDcBlocking_  IndexOptions=Index vector (dialog)  Indices=1  OutputSizes=1
  Data Store Write1 : DataStoreWrite  DataStoreName=oPitch  DataStoreElements=oPitch.oIsr_.oParam_.fAFluxMagnitude_  IndexOptions=Index vector (dialog)  Indices=1  OutputSizes=1
  Data Store Write2 : DataStoreWrite  DataStoreName=oPitch  DataStoreElements=oPitch.oIsr_.oParam_.fALoopfilter2_  IndexOptions=Index vector (dialog)  Indices=1  OutputSizes=1
  Data Store Write3 : DataStoreWrite  DataStoreName=oPitch  DataStoreElements=oPitch.oMot_.oParam_.fObserverLoopFilterBandwidthHz_  IndexOptions=Index vector (dialog)  Indices=1  OutputSizes=1
  Data Store Write4 : DataStoreWrite  DataStoreName=oPitch  DataStoreElements=oPitch.oIsr_.oParam_.fAOmegaFilter2_  IndexOptions=Index vector (dialog)  Indices=1  OutputSizes=1
  Data Store Write5 : DataStoreWrite  DataStoreName=oPitch  DataStoreElements=oPitch.oMot_.oParam_.fAOmegaXfilter2_  IndexOptions=Index vector (dialog)  Indices=1  OutputSizes=1
  Data Store Write6 : DataStoreWrite  DataStoreName=oPitch  DataStoreElements=oPitch.oIsr_.oParam_.oPiDataPll2_.oParameter_.fKp_  IndexOptions=Index vector (dialog)  Indices=1  OutputSizes=1
  Divide{,1,3..4} (4 alike) : Product  Inputs=**
  Divide2 : Product  Inputs=***
  Divide5 : Product  Inputs=*/
  GreaterThan : RelationalOperator  Operator=<  OutDataTypeStr=boolean  RndMeth=Simplest
  Saturation{,1..4} (5 alike) : Saturate  UpperLimit=1.0  LowerLimit=1e-6
  Switch : Switch  Criteria=u2 > Threshold
  wires:
  Divide5/1 -> Data Store Write6/1
  Constant7/1 -> Divide5/1
  Saturation4/1 -> Data Store Write5/1
  oIsr_.oParam_.fControlLoopDt_/1 -> Divide/1, Divide1/1, Divide3/1, Divide2/2, Divide5/2, Divide4/1
  Divide4/1 -> Saturation4/1
  Constant6/1 -> Divide4/2
  Saturation3/1 -> Data Store Write4/1
  Divide3/1 -> Saturation3/1
  Constant5/1 -> Divide3/2
  Switch/1 -> Data Store Write3/1, Divide2/1
  Constant3/1 -> Switch/1
  GreaterThan/1 -> Switch/2
  Constant4/1 -> GreaterThan/2
  fObserverLoopFilterBandwidthHz_/1 -> Switch/3, GreaterThan/1
  Divide2/1 -> Saturation2/1
  Saturation2/1 -> Data Store Write2/1
  Constant2/1 -> Divide2/3
  Divide1/1 -> Saturation1/1
  Saturation1/1 -> Data Store Write1/1
  Constant1/1 -> Divide1/2
  Saturation/1 -> Data Store Write/1
  Divide/1 -> Saturation/1
  Constant/1 -> Divide/2

== system Target_Control_System/Target_Control_System/Simulation Controls/Simulation Data Store Initialization/setupObserverForPosSensor(&oTilt)/softwareIirFilterInitialize() ==
  fFreq3db : Inport
  fControlLoopDt_ : Inport  Port=2  OutDataTypeStr=single
  Constant : Constant  OutDataTypeStr=single  SampleTime=-1
  Constant1 : Constant  Value=0  OutDataTypeStr=single  SampleTime=-1
  Constant2 : Constant  OutDataTypeStr=single  SampleTime=-1
  Data Store Write : DataStoreWrite  DataStoreName=oTilt  DataStoreElements=oTilt.oMot_.oState_.oPosSensor_.oInputSensorSpeedFilter_.afConstantsA_.h0  IndexOptions=Index vector (dialog)  Indices=1  OutputSizes=1
  Data Store Write1 : DataStoreWrite  DataStoreName=oTilt  DataStoreElements=oTilt.oMot_.oState_.oPosSensor_.oInputSensorSpeedFilter_.afConstantsA_.h1  IndexOptions=Index vector (dialog)  Indices=1  OutputSizes=1
  Data Store Write10 : DataStoreWrite  DataStoreName=oTilt  DataStoreElements=oTilt.oMot_.oState_.oPosSensor_.oInputSensorSpeedFilter_.fFilterOutput_  IndexOptions=Index vector (dialog)  Indices=1  OutputSizes=1
  Data Store Write2 : DataStoreWrite  DataStoreName=oTilt  DataStoreElements=oTilt.oMot_.oState_.oPosSensor_.oInputSensorSpeedFilter_.afConstantsA_.h2  IndexOptions=Index vector (dialog)  Indices=1  OutputSizes=1
  Data Store Write3 : DataStoreWrite  DataStoreName=oTilt  DataStoreElements=oTilt.oMot_.oState_.oPosSensor_.oInputSensorSpeedFilter_.afConstantsB_.h2  IndexOptions=Index vector (dialog)  Indices=1  OutputSizes=1
  Data Store Write4 : DataStoreWrite  DataStoreName=oTilt  DataStoreElements=oTilt.oMot_.oState_.oPosSensor_.oInputSensorSpeedFilter_.afConstantsB_.h1  IndexOptions=Index vector (dialog)  Indices=1  OutputSizes=1
  Data Store Write5 : DataStoreWrite  DataStoreName=oTilt  DataStoreElements=oTilt.oMot_.oState_.oPosSensor_.oInputSensorSpeedFilter_.afConstantsB_.h0  IndexOptions=Index vector (dialog)  Indices=1  OutputSizes=1
  Data Store Write6 : DataStoreWrite  DataStoreName=oTilt  DataStoreElements=oTilt.oMot_.oState_.oPosSensor_.oInputSensorSpeedFilter_.afPreviousInputs_.h0  IndexOptions=Index vector (dialog)  Indices=1  OutputSizes=1
  Data Store Write7 : DataStoreWrite  DataStoreName=oTilt  DataStoreElements=oTilt.oMot_.oState_.oPosSensor_.oInputSensorSpeedFilter_.afPreviousInputs_.h1  IndexOptions=Index vector (dialog)  Indices=1  OutputSizes=1
  Data Store Write8 : DataStoreWrite  DataStoreName=oTilt  DataStoreElements=oTilt.oMot_.oState_.oPosSensor_.oInputSensorSpeedFilter_.afPreviousOutputs_.h0  IndexOptions=Index vector (dialog)  Indices=1  OutputSizes=1
  Data Store Write9 : DataStoreWrite  DataStoreName=oTilt  DataStoreElements=oTilt.oMot_.oState_.oPosSensor_.oInputSensorSpeedFilter_.afPreviousOutputs_.h1  IndexOptions=Index vector (dialog)  Indices=1  OutputSizes=1
  Data Type Conversion{,1..4} (5 alike) : DataTypeConversion  OutDataTypeStr=single
  Demux : Demux  Outputs=6
  Divide : Product  Inputs=*/  OutDataTypeStr=single
  Divide1 : Product  Inputs=*/  OutDataTypeStr=single
  computeCoefficientsButter() : Subsystem
  fActualFrequencyHz : Outport
  wires:
  Constant2/1 -> Divide1/1
  fControlLoopDt_/1 -> Divide1/2
  Divide1/1 -> computeCoefficientsButter()/2(dSampleFrequencyHz)
  Data Type Conversion4/1 -> Data Store Write2/1
  Data Type Conversion3/1 -> Data Store Write1/1
  Data Type Conversion2/1 -> Data Store Write3/1
  Data Type Conversion/1 -> Data Store Write4/1
  Data Type Conversion1/1 -> Data Store Write5/1
  Constant1/1 -> Data Store Write6/1, Data Store Write7/1, Data Store Write9/1, Data Store Write10/1, Data Store Write8/1
  Demux/1 -> Data Type Conversion1/1
  Demux/2 -> Data Type Conversion/1
  Constant/1 -> Divide/1
  Divide/1 -> Data Store Write/1
  Demux/4 -> Divide/2
  Demux/3 -> Data Type Conversion2/1
  Demux/5 -> Data Type Conversion3/1
  Demux/6 -> Data Type Conversion4/1
  computeCoefficientsButter()/1(dpOutArray) -> Demux/1
  fFreq3db/1 -> computeCoefficientsButter()/1(fCutoffFrequencyHz)
  computeCoefficientsButter()/2(fFreq3db) -> fActualFrequencyHz/1

== system Target_Control_System/Target_Control_System/Simulation Controls/Simulation Data Store Initialization/setupPwm(&oTilt)/setPwmFrequencyApplication()_tilt ==
  fPwmFreqKhz_ : Inport
  fMotorAccelerationStage1Bandwidth_ : Inport  Port=2
  fFilterBandwidthForSpeedControlIqRef_ : Inport  Port=3
  Data Store Read : DataStoreRead  Priority=5  DataStoreName=oProp  DataStoreElements=oProp.oIsr_.oParam_.fControlLoopDt_  IndexOptions=Index vector (dialog)  Indices=1  OutputSizes=1
  Data Store Read1 : DataStoreRead  Priority=5  DataStoreName=oTilt  DataStoreElements=oTilt.oMot_.oParam_.fObserverLoopFilterBandwidthHz_  IndexOptions=Index vector (dialog)  Indices=1  OutputSizes=1
  Data Store Write : DataStoreWrite  Priority=5  DataStoreName=oTilt  DataStoreElements=oTilt.oIsr_.oParam_.fControlLoopDt_  IndexOptions=Index vector (dialog)  Indices=1  OutputSizes=1
  Data Store Write1 : DataStoreWrite  Priority=5  DataStoreName=oTilt  DataStoreElements=oTilt.oMot_.oParam_.fIntControlLoopDt_  IndexOptions=Index vector (dialog)  Indices=1  OutputSizes=1
  Gain : Gain  Priority=5  Gain=4  OutDataTypeStr=single
  setPwmFrequency()_tilt : Subsystem  Priority=1  TreatAsAtomicUnit=on
  updateObserver()_tilt : Subsystem  Priority=10  TreatAsAtomicUnit=on
  wires:
  Gain/1 -> Data Store Write/1, Data Store Write1/1, updateObserver()_tilt/1(oIsr_.oParam_.fControlLoopDt_)
  Data Store Read/1 -> Gain/1
  Data Store Read1/1 -> updateObserver()_tilt/2(fObserverLoopFilterBandwidthHz_)
  fFilterBandwidthForSpeedControlIqRef_/1 -> setPwmFrequency()_tilt/3(fFilterBandwidthForSpeedControlIqRef_)
  fMotorAccelerationStage1Bandwidth_/1 -> setPwmFrequency()_tilt/2(fMotorAccelerationStage1Bandwidth_)
  fPwmFreqKhz_/1 -> setPwmFrequency()_tilt/1(fPwmFreqKhz_)

== system Target_Control_System/Target_Control_System/Simulation Controls/Simulation Data Store Initialization/setupPwm()/setPwmFrequencyApplication()_pitch ==
  fPwmFreqKhz_ : Inport
  fMotorAccelerationStage1Bandwidth_ : Inport  Port=2
  fFilterBandwidthForSpeedControlIqRef_ : Inport  Port=3
  Data Store Read : DataStoreRead  Priority=5  DataStoreName=oProp  DataStoreElements=oProp.oIsr_.oParam_.fControlLoopDt_  IndexOptions=Index vector (dialog)  Indices=1  OutputSizes=1
  Data Store Read1 : DataStoreRead  Priority=5  DataStoreName=oPitch  DataStoreElements=oPitch.oMot_.oParam_.fObserverLoopFilterBandwidthHz_  IndexOptions=Index vector (dialog)  Indices=1  OutputSizes=1
  Data Store Write : DataStoreWrite  Priority=5  DataStoreName=oPitch  DataStoreElements=oPitch.oIsr_.oParam_.fControlLoopDt_  IndexOptions=Index vector (dialog)  Indices=1  OutputSizes=1
  Data Store Write1 : DataStoreWrite  Priority=5  DataStoreName=oPitch  DataStoreElements=oPitch.oMot_.oParam_.fIntControlLoopDt_  IndexOptions=Index vector (dialog)  Indices=1  OutputSizes=1
  Gain : Gain  Priority=5  Gain=4  OutDataTypeStr=single
  setPwmFrequency()_pitch : Subsystem  Priority=1  TreatAsAtomicUnit=on
  updateObserver()_pitch : Subsystem  Priority=10  TreatAsAtomicUnit=on
  wires:
  Gain/1 -> Data Store Write/1, Data Store Write1/1, updateObserver()_pitch/1(oIsr_.oParam_.fControlLoopDt_)
  Data Store Read/1 -> Gain/1
  Data Store Read1/1 -> updateObserver()_pitch/2(fObserverLoopFilterBandwidthHz_)
  fFilterBandwidthForSpeedControlIqRef_/1 -> setPwmFrequency()_pitch/3(fFilterBandwidthForSpeedControlIqRef_)
  fMotorAccelerationStage1Bandwidth_/1 -> setPwmFrequency()_pitch/2(fMotorAccelerationStage1Bandwidth_)
  fPwmFreqKhz_/1 -> setPwmFrequency()_pitch/1(fPwmFreqKhz_)

== system Target_Control_System/Target_Control_System/Simulation Controls/Simulation Data Store Initialization/updateServoObserver(&oTilt)/updateServoObserver() ==
  oIsr_.oParam_.fControlLoopDt_ : Inport  OutDataTypeStr=single
  fOmegaEDifferentiatorBandwidthHz_ : Inport  Port=2  OutDataTypeStr=single
  Constant : Constant  OutDataTypeStr=single  SampleTime=-1
  Data Store Write : DataStoreWrite  DataStoreName=oTilt  DataStoreElements=oTilt.oMot_.oState_.oPosSensor_.fOmegaEDifferentiatorBandwidthHz_  IndexOptions=Index vector (dialog)  Indices=1  OutputSizes=1
  Divide : Product  Inputs=*/  OutDataTypeStr=single
  softwareIirFilterInitialize() : Subsystem  TreatAsAtomicUnit=on
  wires:
  fOmegaEDifferentiatorBandwidthHz_/1 -> softwareIirFilterInitialize()/1(fFreq3db)
  Divide/1 -> softwareIirFilterInitialize()/2(fFreqSample)
  oIsr_.oParam_.fControlLoopDt_/1 -> Divide/2
  softwareIirFilterInitialize()/1(fActualFrequencyHz) -> Data Store Write/1
  Constant/1 -> Divide/1

== system Target_Control_System/Target_Control_System/Simulation Controls/Simulation Data Store Initialization/updateServoObserver()/updateServoObserver()_pitch ==
  oIsr_.oParam_.fControlLoopDt_ : Inport  OutDataTypeStr=single
  fOmegaEDifferentiatorBandwidthHz_ : Inport  Port=2  OutDataTypeStr=single
  Constant : Constant  OutDataTypeStr=single  SampleTime=-1
  Data Store Write : DataStoreWrite  DataStoreName=oPitch  DataStoreElements=oPitch.oMot_.oState_.oPosSensor_.fOmegaEDifferentiatorBandwidthHz_  IndexOptions=Index vector (dialog)  Indices=1  OutputSizes=1
  Divide : Product  Inputs=*/  OutDataTypeStr=single
  softwareIirFilterInitialize() : Subsystem  TreatAsAtomicUnit=on
  wires:
  fOmegaEDifferentiatorBandwidthHz_/1 -> softwareIirFilterInitialize()/1(fFreq3db)
  Divide/1 -> softwareIirFilterInitialize()/2(fFreqSample)
  oIsr_.oParam_.fControlLoopDt_/1 -> Divide/2
  softwareIirFilterInitialize()/1(fActualFrequencyHz) -> Data Store Write/1
  Constant/1 -> Divide/1

== system Target_Control_System/Target_Control_System/Simulation Controls/pitchMotor/Apply Simulation Setpoints/Set Current ==
  Current Setpoint for Simulation : Inport
  Enable : EnablePort
  Data Store Write1 : DataStoreWrite  DataStoreName=oPitch  DataStoreElements=oPitch.oMot_.oIn_.fIqSetpoint_  IndexOptions=Index vector (dialog)  Indices=1  OutputSizes=1
  wires:
  Current Setpoint for Simulation/1 -> Data Store Write1/1

== system Target_Control_System/Target_Control_System/Simulation Controls/pitchMotor/Apply Simulation Setpoints/Set Position ==
  Position Setpoint for Simulation : Inport
  Enable : EnablePort
  Data Store Write3 : DataStoreWrite  DataStoreName=oPitch  DataStoreElements=oPitch.oMot_.oIn_.fPosSetpoint_  IndexOptions=Index vector (dialog)  Indices=1  OutputSizes=1
  wires:
  Position Setpoint for Simulation/1 -> Data Store Write3/1

== system Target_Control_System/Target_Control_System/Simulation Controls/pitchMotor/Apply Simulation Setpoints/Set Speed ==
  Speed Setpoint for Simulation : Inport
  Enable : EnablePort
  Data Store Write2 : DataStoreWrite  DataStoreName=oPitch  DataStoreElements=oPitch.oMot_.oIn_.fRpmSetpoint_  IndexOptions=Index vector (dialog)  Indices=1  OutputSizes=1
  wires:
  Speed Setpoint for Simulation/1 -> Data Store Write2/1

== system Target_Control_System/Target_Control_System/Simulation Controls/pitchMotor/Initialize controller/Set Current Controller ==
  Enable : EnablePort
  Bus Assignment : BusAssignment  AssignedSignals=oMot_.oOut_.uiCurrentControllerActive_,oMot_.oState_.uiSpeedControllerActive_,oMot_.oState_.oPosSensor_.iPosControlEnabled_,oMot_.oParam_.uiTorqueMirroringActive_
  Constant14 : Constant  Value=0  OutDataTypeStr=int32  SampleTime=-1
  Constant16 : Constant  Value=0  OutDataTypeStr=uint32  SampleTime=-1
  Constant5 : Constant  OutDataTypeStr=uint32  SampleTime=-1
  Constant7 : Constant  Value=0  OutDataTypeStr=uint32  SampleTime=-1
  Data Store Read : DataStoreRead  DataStoreName=oPitch  IndexOptions=Index vector (dialog)  Indices=1  OutputSizes=1
  Data Store Write5 : DataStoreWrite  DataStoreName=oPitch  IndexOptions=Index vector (dialog)  Indices=1  OutputSizes=1
  wires:
  Constant7/1 -> Bus Assignment/3
  Constant16/1 -> Bus Assignment/5
  Constant14/1 -> Bus Assignment/4
  Data Store Read/1 -> Bus Assignment/1
  Constant5/1 -> Bus Assignment/2
  Bus Assignment/1 -> Data Store Write5/1

== system Target_Control_System/Target_Control_System/Simulation Controls/pitchMotor/Initialize controller/Set Position Controller ==
  Enable : EnablePort
  Bus Assignment2 : BusAssignment  AssignedSignals=oMot_.oOut_.uiCurrentControllerActive_,oMot_.oState_.uiSpeedControllerActive_,oMot_.oState_.oPosSensor_.iPosControlEnabled_,oMot_.oParam_.uiTorqueMirroringActive_
  Constant11 : Constant  OutDataTypeStr=uint32  SampleTime=-1
  Constant12 : Constant  Value=0  OutDataTypeStr=uint32  SampleTime=-1
  Constant9 : Constant  OutDataTypeStr=int32  SampleTime=-1
  Data Store Read : DataStoreRead  DataStoreName=oPitch  IndexOptions=Index vector (dialog)  Indices=1  OutputSizes=1
  Data Store Write2 : DataStoreWrite  DataStoreName=oPitch  IndexOptions=Index vector (dialog)  Indices=1  OutputSizes=1
  wires:
  Constant9/1 -> Bus Assignment2/4
  Bus Assignment2/1 -> Data Store Write2/1
  Data Store Read/1 -> Bus Assignment2/1
  Constant11/1 -> Bus Assignment2/2, Bus Assignment2/3
  Constant12/1 -> Bus Assignment2/5

== system Target_Control_System/Target_Control_System/Simulation Controls/pitchMotor/Initialize controller/Set Speed Controller ==
  Enable : EnablePort
  Bus Assignment1 : BusAssignment  AssignedSignals=oMot_.oOut_.uiCurrentControllerActive_,oMot_.oState_.uiSpeedControllerActive_,oMot_.oState_.oPosSensor_.iPosControlEnabled_,oMot_.oParam_.uiTorqueMirroringActive_
  Constant10 : Constant  Value=0  OutDataTypeStr=int32  SampleTime=-1
  Constant2 : Constant  OutDataTypeStr=uint32  SampleTime=-1
  Constant4 : Constant  Value=0  OutDataTypeStr=uint32  SampleTime=-1
  Data Store Read1 : DataStoreRead  DataStoreName=oPitch  IndexOptions=Index vector (dialog)  Indices=1  OutputSizes=1
  Data Store Write3 : DataStoreWrite  DataStoreName=oPitch  IndexOptions=Index vector (dialog)  Indices=1  OutputSizes=1
  wires:
  Bus Assignment1/1 -> Data Store Write3/1
  Constant10/1 -> Bus Assignment1/4
  Constant4/1 -> Bus Assignment1/5
  Data Store Read1/1 -> Bus Assignment1/1
  Constant2/1 -> Bus Assignment1/2, Bus Assignment1/3

== system Target_Control_System/Target_Control_System/Simulation Controls/tiltMotor/Apply Simulation Setpoints/Set Current ==
  Current Setpoint for Simulation : Inport
  Enable : EnablePort
  Data Store Write2 : DataStoreWrite  DataStoreName=oTilt  DataStoreElements=oTilt.oMot_.oIn_.fIqSetpoint_  IndexOptions=Index vector (dialog)  Indices=1  OutputSizes=1
  wires:
  Current Setpoint for Simulation/1 -> Data Store Write2/1

== system Target_Control_System/Target_Control_System/Simulation Controls/tiltMotor/Apply Simulation Setpoints/Set Position ==
  Position Setpoint for Simulation : Inport
  Enable : EnablePort
  Data Store Write1 : DataStoreWrite  DataStoreName=oTilt  DataStoreElements=oTilt.oMot_.oIn_.fPosSetpoint_  IndexOptions=Index vector (dialog)  Indices=1  OutputSizes=1
  wires:
  Position Setpoint for Simulation/1 -> Data Store Write1/1

== system Target_Control_System/Target_Control_System/Simulation Controls/tiltMotor/Apply Simulation Setpoints/Set Speed ==
  Speed Setpoint for Simulation : Inport
  Enable : EnablePort
  Data Store Write1 : DataStoreWrite  DataStoreName=oTilt  DataStoreElements=oTilt.oMot_.oIn_.fRpmSetpoint_  IndexOptions=Index vector (dialog)  Indices=1  OutputSizes=1
  wires:
  Speed Setpoint for Simulation/1 -> Data Store Write1/1

== system Target_Control_System/Target_Control_System/Simulation Controls/tiltMotor/Initialize controller/Set Current Controller ==
  Enable : EnablePort
  Bus Assignment : BusAssignment  AssignedSignals=oMot_.oOut_.uiCurrentControllerActive_,oMot_.oState_.uiSpeedControllerActive_,oMot_.oState_.oPosSensor_.iPosControlEnabled_,oMot_.oParam_.uiTorqueMirroringActive_
  Constant14 : Constant  Value=0  OutDataTypeStr=int32  SampleTime=-1
  Constant16 : Constant  Value=0  OutDataTypeStr=uint32  SampleTime=-1
  Constant5 : Constant  OutDataTypeStr=uint32  SampleTime=-1
  Constant7 : Constant  Value=0  OutDataTypeStr=uint32  SampleTime=-1
  Data Store Read : DataStoreRead  DataStoreName=oTilt  IndexOptions=Index vector (dialog)  Indices=1  OutputSizes=1
  Data Store Write5 : DataStoreWrite  DataStoreName=oTilt  IndexOptions=Index vector (dialog)  Indices=1  OutputSizes=1
  wires:
  Constant7/1 -> Bus Assignment/3
  Constant16/1 -> Bus Assignment/5
  Constant14/1 -> Bus Assignment/4
  Data Store Read/1 -> Bus Assignment/1
  Constant5/1 -> Bus Assignment/2
  Bus Assignment/1 -> Data Store Write5/1

== system Target_Control_System/Target_Control_System/Simulation Controls/tiltMotor/Initialize controller/Set Position Controller ==
  Enable : EnablePort
  Bus Assignment2 : BusAssignment  AssignedSignals=oMot_.oOut_.uiCurrentControllerActive_,oMot_.oState_.uiSpeedControllerActive_,oMot_.oState_.oPosSensor_.iPosControlEnabled_,oMot_.oParam_.uiTorqueMirroringActive_
  Constant11 : Constant  OutDataTypeStr=uint32  SampleTime=-1
  Constant12 : Constant  Value=0  OutDataTypeStr=uint32  SampleTime=-1
  Constant9 : Constant  OutDataTypeStr=int32  SampleTime=-1
  Data Store Read : DataStoreRead  DataStoreName=oTilt  IndexOptions=Index vector (dialog)  Indices=1  OutputSizes=1
  Data Store Write2 : DataStoreWrite  DataStoreName=oTilt  IndexOptions=Index vector (dialog)  Indices=1  OutputSizes=1
  wires:
  Constant9/1 -> Bus Assignment2/4
  Bus Assignment2/1 -> Data Store Write2/1
  Data Store Read/1 -> Bus Assignment2/1
  Constant11/1 -> Bus Assignment2/2, Bus Assignment2/3
  Constant12/1 -> Bus Assignment2/5

== system Target_Control_System/Target_Control_System/Simulation Controls/tiltMotor/Initialize controller/Set Speed Controller ==
  Enable : EnablePort
  Bus Assignment1 : BusAssignment  AssignedSignals=oMot_.oOut_.uiCurrentControllerActive_,oMot_.oState_.uiSpeedControllerActive_,oMot_.oState_.oPosSensor_.iPosControlEnabled_,oMot_.oParam_.uiTorqueMirroringActive_
  Constant10 : Constant  Value=0  OutDataTypeStr=int32  SampleTime=-1
  Constant2 : Constant  OutDataTypeStr=uint32  SampleTime=-1
  Constant4 : Constant  Value=0  OutDataTypeStr=uint32  SampleTime=-1
  Data Store Read1 : DataStoreRead  DataStoreName=oTilt  IndexOptions=Index vector (dialog)  Indices=1  OutputSizes=1
  Data Store Write3 : DataStoreWrite  DataStoreName=oTilt  IndexOptions=Index vector (dialog)  Indices=1  OutputSizes=1
  wires:
  Bus Assignment1/1 -> Data Store Write3/1
  Constant10/1 -> Bus Assignment1/4
  Constant4/1 -> Bus Assignment1/5
  Data Store Read1/1 -> Bus Assignment1/1
  Constant2/1 -> Bus Assignment1/2, Bus Assignment1/3

== system Target_Control_System/Target_Control_System/InterruptFunction/pitchMotor_dataToMain/Variant Subsystem/VP_leader_follower_postion_copy/Follower Postion Enabled Subsystem ==
  Enable : EnablePort
  System Update : Subsystem  mask(System Update){ShowInLibBrowser=0}
      mask prompts: ShowInLibBrowser "Simulink:masks:CustCodeMaskParam1_MP"
      settings: CopyFcn=cccopyfcn(gcb)  OpenFcn=ccopenfcn('System Update Function')
      mask Help: eval('feval(''rtwprivate'',''rtwhelpview'',''rtw_sys_update_block'')');
      mask Display: disp('System\nUpdate');

== system Target_Control_System/Target_Control_System/InterruptFunction/pitchMotor_dataToMain/Variant Subsystem/VP_leader_follower_postion_copy/Leader Postion Enabled Subsystem ==
  Enable : EnablePort
  System Update : Subsystem  mask(System Update){ShowInLibBrowser=0}
      mask prompts: ShowInLibBrowser "Simulink:masks:CustCodeMaskParam1_MP"
      settings: CopyFcn=cccopyfcn(gcb)  OpenFcn=ccopenfcn('System Update Function')
      mask Help: eval('feval(''rtwprivate'',''rtwhelpview'',''rtw_sys_update_block'')');
      mask Display: disp('System\nUpdate');
